simulink model "DCM"  (R2021b)
settings: Solver=VariableStepAuto  StartTime=0.0  StopTime=2  MaxStep=1e-4  RelTol=1e-3
libraries: spsVoltageMeasurementLib x7, spsSeriesRLCBranchLib x5, spsDiodeLib x3, spsCurrentMeasurementLib x1, spsDCVoltageSourceLib x1, spsIGBTDiodeLib x1, simulink x1, spspowerguiLib x1
settings Model: Creator=ttkl1  LastModifiedBy=Legion

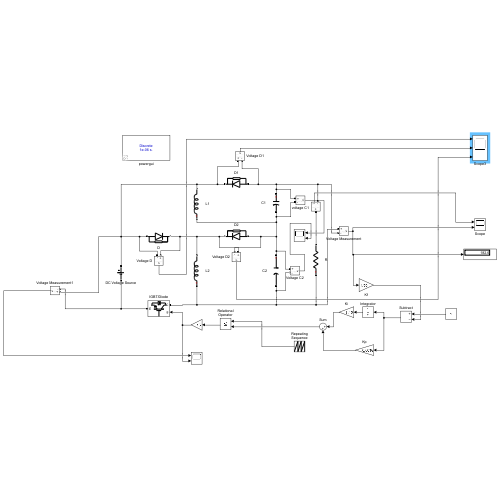
[thumbnail: Simulink's stored preview of the top-level diagram]
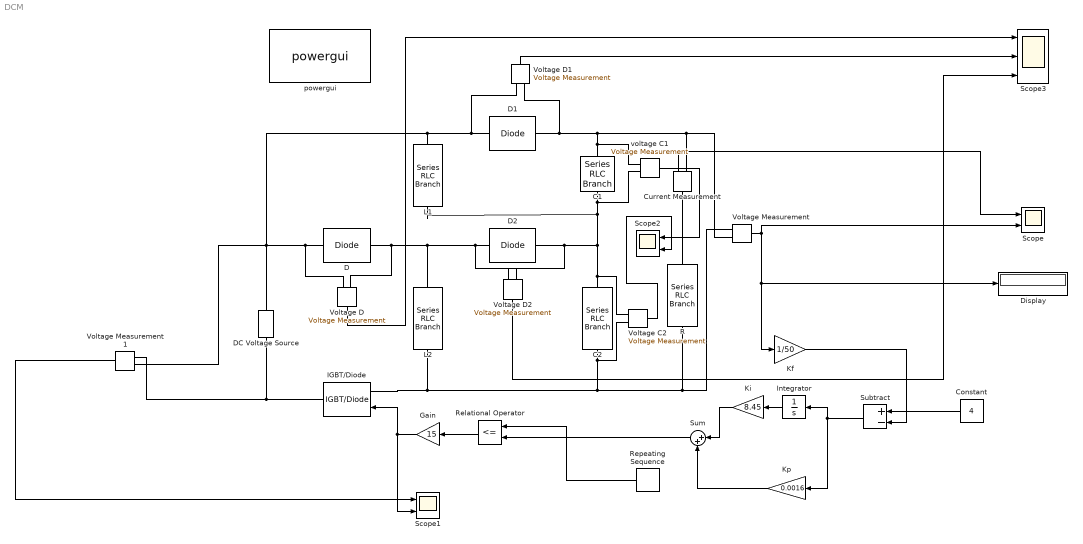
== system DCM ==
  C1 : spsSeriesRLCBranchLib/Series RLC Branch  LConnTagsString=__new0  RConnTagsString=__new0  BranchType=C  Resistance=1  Inductance=1e-3  SetiL0=off  InitialCurrent=0  Capacitance=100e-6  Setx0=off  InitialVoltage=0  Measurements=None
  C2 : spsSeriesRLCBranchLib/Series RLC Branch  LConnTagsString=__new0  RConnTagsString=__new0  BranchType=C  Resistance=1  Inductance=1e-3  SetiL0=off  InitialCurrent=0  Capacitance=100e-6  Setx0=off  InitialVoltage=0  Measurements=None
  Constant : Constant  Value=4
  Current Measurement : spsCurrentMeasurementLib/Current Measurement  PhasorSimulation=off  OutputType=Complex  PSBequivalent=0
  D : spsDiodeLib/Diode  Ron=0.001  Lon=0  Vf=0  IC=0  UseSnubber=0  Rs=500  Cs=250e-9  Measurements=off
  D1 : spsDiodeLib/Diode  Ron=0.001  Lon=0  Vf=0  IC=0  UseSnubber=0  Rs=500  Cs=250e-9  Measurements=off
  D2 : spsDiodeLib/Diode  Ron=0.001  Lon=0  Vf=0  IC=0  UseSnubber=0  Rs=500  Cs=250e-9  Measurements=off
  DC Voltage Source : spsDCVoltageSourceLib/DC Voltage Source  Amplitude=50  Measurements=None
  Display : Display
  Gain : Gain  Gain=15
  IGBT/Diode : spsIGBTDiodeLib/IGBT//Diode  Ron=1e-3  Rs=1e5  Cs=inf  Measurements=off
  Integrator : Integrator
  Kf : Gain  Gain=1/50
  Ki : Gain  Gain=8.45
  Kp : Gain  Gain=0.0016
  L1 : spsSeriesRLCBranchLib/Series RLC Branch  LConnTagsString=__new0  RConnTagsString=__new0  BranchType=L  Resistance=1  Inductance=16e-3  SetiL0=off  InitialCurrent=0  Capacitance=1e-6  Setx0=off  InitialVoltage=0  Measurements=None
  L2 : spsSeriesRLCBranchLib/Series RLC Branch  LConnTagsString=__new0  RConnTagsString=__new0  BranchType=L  Resistance=1  Inductance=3e-3  SetiL0=off  InitialCurrent=0  Capacitance=1e-6  Setx0=off  InitialVoltage=0  Measurements=None
  R : spsSeriesRLCBranchLib/Series RLC Branch  LConnTagsString=__new0  RConnTagsString=__new0  BranchType=R  Resistance=200  Inductance=1e-3  SetiL0=off  InitialCurrent=0  Capacitance=1e-6  Setx0=off  InitialVoltage=0  Measurements=None
  Relational Operator : RelationalOperator  Operator=<=  OutDataTypeStr=boolean  RndMeth=Simplest
  Repeating Sequence : simulink/Sources/Repeating Sequence  rep_seq_t=[0 1/10000]  rep_seq_y=[0 2]
  Scope : Scope  NumInputPorts=2
  Scope1 : Scope  NumInputPorts=2
  Scope2 : Scope  NumInputPorts=2
  Scope3 : Scope  NumInputPorts=3
  Subtract : Sum  Inputs=+-
  Sum : Sum  Inputs=|++
  Voltage C2 : spsVoltageMeasurementLib/Voltage Measurement  PhasorSimulation=off  OutputType=Complex  PSBequivalent=0
  Voltage D : spsVoltageMeasurementLib/Voltage Measurement  PhasorSimulation=off  OutputType=Complex  PSBequivalent=0
  Voltage D1 : spsVoltageMeasurementLib/Voltage Measurement  PhasorSimulation=off  OutputType=Complex  PSBequivalent=0
  Voltage D2 : spsVoltageMeasurementLib/Voltage Measurement  PhasorSimulation=off  OutputType=Complex  PSBequivalent=0
  Voltage Measurement : spsVoltageMeasurementLib/Voltage Measurement  PhasorSimulation=off  OutputType=Complex  PSBequivalent=0
  Voltage Measurement1 : spsVoltageMeasurementLib/Voltage Measurement  PhasorSimulation=off  OutputType=Complex  PSBequivalent=0
  powergui : spspowerguiLib/powergui  Priority=1  SimulationMode=Discrete  SampleTime=1e-6  frequency=60  Iterations=50  frequencyindice=0  Pbase=100e6  ErrMax=1e-4  UnitsV=kV  UnitsW=MW  buscounter=0  FunctionMessages=off  echomessages=off  EnableUseOfTLC=off  CurrentSourceSwitches=off  DisableSnubberDevices=off  DisableRonSwitches=off  DisableVfSwitches=off  DisplayEquations=off  AutomaticDiscreteSolvers=off  SolverType=Tustin/Backward Euler (TBE)  Interpol=off  ExternalGateDelay=off  methode=off  Ts=100  x0status=blocks  SPID=on  SwTol=0  HookPort=off  NonlinearTolerance=1e-4  nMaxIteration=100  ContinueOnMaxIteration=off  RestoreLinks=warning  ResistiveCurrentMeasurement=off  Frange=[0:2:500]  Ylog=off  Xlog=on  ShowGrid=off  save=off  variable=ZData  structure=0  ZoomFFT=off  StartTime=0.0  cycles=1  DisplayStyle=1  fundamental=60  FreqAxis=off  MaxFrequency=1000  frequencyindicesteady=1  RmsSteady=1  display=off
  voltage C1 : spsVoltageMeasurementLib/Voltage Measurement  PhasorSimulation=off  OutputType=Complex  PSBequivalent=0
  wires:
  Voltage Measurement/1 -> Kf/1, Display/1, Scope/2
  Relational Operator/1 -> Gain/1
  Ki/1 -> Sum/1
  Integrator/1 -> Ki/1
  Subtract/1 -> Kp/1, Integrator/1
  Kf/1 -> Subtract/2
  Kp/1 -> Sum/2
  Voltage Measurement1/1 -> Scope1/1
  Sum/1 -> Relational Operator/2
  Repeating Sequence/1 -> Relational Operator/1
  Current Measurement/1 -> Scope/1
  Voltage C2/1 -> Scope2/2
  voltage C1/1 -> Scope2/1
  Gain/1 -> IGBT/Diode/1, Scope1/2
  Constant/1 -> Subtract/1
  Voltage D2/1 -> Scope3/3
  Voltage D1/1 -> Scope3/2
  Voltage D/1 -> Scope3/1
  connections:
  L1/LConn1 -- C1/RConn1 -- voltage C1/LConn2 -- Voltage D2/LConn2 -- D2/LConn1 -- C2/LConn1 -- Voltage C2/LConn1
  L2/LConn1 -- IGBT/Diode/LConn1 -- R/LConn1 -- Voltage Measurement/LConn1 -- C2/RConn1 -- Voltage C2/LConn2
  Voltage Measurement/LConn2 -- Current Measurement/RConn1 -- Voltage D1/LConn2 -- D1/LConn1 -- voltage C1/LConn1 -- C1/LConn1
  L2/RConn1 -- Voltage D/LConn1 -- D/RConn1 -- Voltage D2/LConn1 -- D2/RConn1
  DC Voltage Source/LConn1 -- Voltage Measurement1/LConn2 -- IGBT/Diode/RConn1
  D1/RConn1 -- Voltage Measurement1/LConn1 -- DC Voltage Source/RConn1 -- Voltage D/LConn2 -- D/LConn1 -- L1/RConn1 -- Voltage D1/LConn1
  Current Measurement/LConn1 -- R/RConn1
